simulink model "sim_punto_2"  (R2021b)
settings: Solver=VariableStepAuto  StartTime=0.0  StopTime=10.0  RelTol=1e-3
values from neighbouring files (symbols this model uses):
  A = [0 1 0 0 0 0 0 0 0 0 0 0 ... (first row only)    [punto2.m]
  B = [0; 0; 0; 0; 0; 0; 0; 0; 0; 0; 0; 1]    [punto2.m]
  C = [1 0 0 0 0 0 0 0 0 0 0 0]    [punto2.m]
  C_states = eye(12)    [punto2.m]
  D_states = [0 0 0 0 0 0 0 0 0 0 0 0]'    [punto2.m]
  N = 1    [punto2.m]
  Q = [1+q 0 0 0 0 0 0 0 0 0 0 0 ... (first row only)    [punto2.m]
  R = r    (= 1e-05)    [punto2.m]
  S = Pr    [punto2.m]
  Ts = 0.1    [punto2.m]
  U_max = 15    [punto2.m]
  U_min = -15    [punto2.m]
  Ubar = inv(g)*Ybar    [punto2.m]
  x0 = [0 0 0 0 0 0 0 0 0 0 0 0]'    [punto2.m]
  Xbar = -inv(A) * B * Ubar    [punto2.m]
  Xbar_disc = (eye(12)- A)^-1*B*Ubar    [punto2.m]
undefined symbols (not defined in the file or in its folder): K_disc, mympc
settings Model: Creator=danie  LastModifiedBy=danie

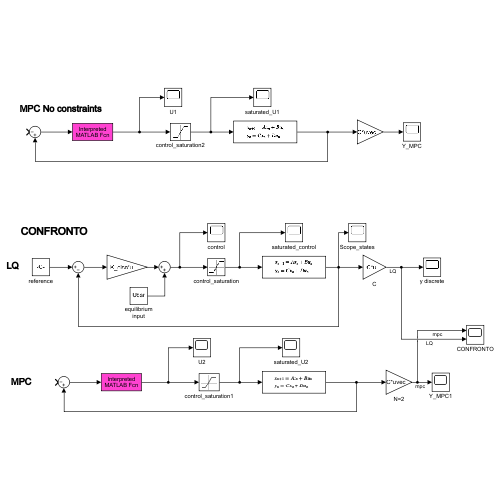
[thumbnail: Simulink's stored preview of the top-level diagram]
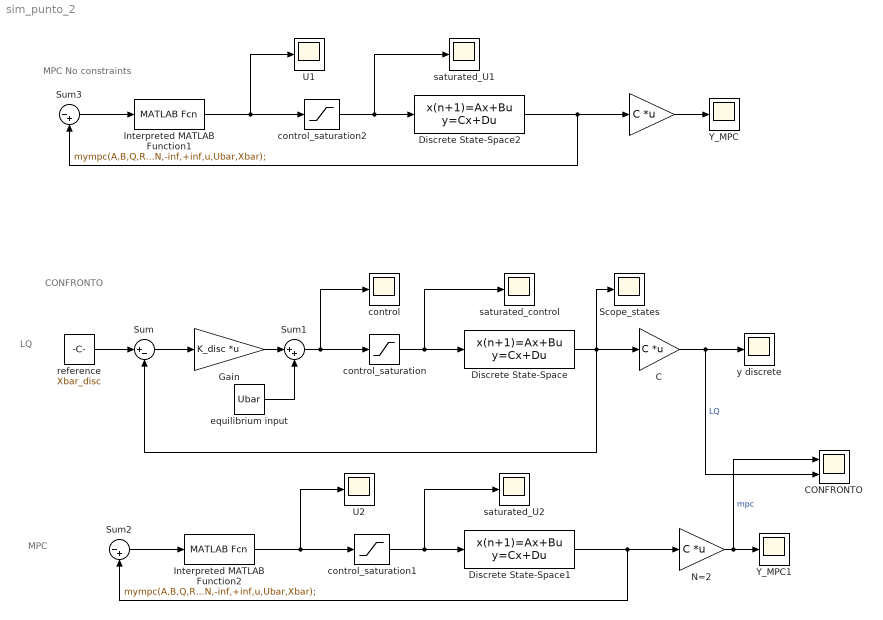
== system sim_punto_2 ==
  note: LQ
  note: CONFRONTO
  note: MPC
  note: MPC No constraints
  " " : Gain  Gain=C  Multiplication=Matrix(K*u) (u vector)
  C : Gain  Gain=C  Multiplication=Matrix(K*u)
  CONFRONTO : Scope  NumInputPorts=2
  Discrete State-Space : DiscreteStateSpace  A=A  B=B  C=C_states  D=D_states  SampleTime=Ts
  Discrete State-Space1 : DiscreteStateSpace  A=A  B=B  C=C_states  D=D_states  InitialCondition=x0  SampleTime=Ts
  Discrete State-Space2 : DiscreteStateSpace  A=A  B=B  C=C_states  D=D_states  InitialCondition=x0  SampleTime=Ts
  Gain : Gain  Gain=K_disc  Multiplication=Matrix(K*u)
  Interpreted MATLAB Function1 : MATLABFcn  MATLABFcn=mympc(A,B,Q,R,S,N,-inf,+inf,u,Ubar,Xbar);  OutputDimensions=1
  Interpreted MATLAB Function2 : MATLABFcn  MATLABFcn=mympc(A,B,Q,R,S,N,-inf,+inf,u,Ubar,Xbar);  OutputDimensions=1
  N=2 : Gain  Gain=C  Multiplication=Matrix(K*u) (u vector)
  Scope_states : Scope
  Sum : Sum  Inputs=|+-
  Sum1 : Sum  Inputs=|++
  Sum2 : Sum  Inputs=|-+
  Sum3 : Sum  Inputs=|-+
  U1 : Scope
  U2 : Scope
  Y_MPC : Scope
  Y_MPC1 : Scope
  control : Scope
  control_saturation : Saturate  UpperLimit=U_max  LowerLimit=U_min
  control_saturation1 : Saturate  UpperLimit=U_max  LowerLimit=U_min
  control_saturation2 : Saturate  UpperLimit=U_max  LowerLimit=U_min
  equilibrium input : Constant  Value=Ubar
  reference : Constant  Value=Xbar_disc
  saturated_U1 : Scope
  saturated_U2 : Scope
  saturated_control : Scope
  y discrete : Scope
  wires:
  " "/1 -> Y_MPC/1
  Sum3/1 -> Interpreted MATLAB Function1/1
  Interpreted MATLAB Function1/1 -> control_saturation2/1, U1/1
  control_saturation2/1 -> saturated_U1/1, Discrete State-Space2/1
  Discrete State-Space2/1 -> Sum3/2, " "/1
  Sum/1 -> Gain/1
  Sum1/1 -> control/1, control_saturation/1
  C/1 -> CONFRONTO/2, y discrete/1  "LQ"
  reference/1 -> Sum/1
  Discrete State-Space/1 -> C/1, Scope_states/1, Sum/2
  control_saturation/1 -> Discrete State-Space/1, saturated_control/1
  Gain/1 -> Sum1/1
  equilibrium input/1 -> Sum1/2
  N=2/1 -> CONFRONTO/1, Y_MPC1/1  "mpc"
  Discrete State-Space1/1 -> Sum2/2, N=2/1
  control_saturation1/1 -> saturated_U2/1, Discrete State-Space1/1
  Interpreted MATLAB Function2/1 -> control_saturation1/1, U2/1
  Sum2/1 -> Interpreted MATLAB Function2/1
